simulink model "Sim_V1_scaling"  (R2018a)
settings: Solver=FixedStepAuto  StartTime=0.0  StopTime=tend  FixedStep=dt  MinStep=1e-3  RelTol=1e-3
values from neighbouring files (symbols this model uses):
  aref0 = a0+c*v0    [Init_Plots_Paper_V12.m]    (also in Init_Plots_Paper_V12_compare_high_low_fb.m; Init_Plots_Paper_V12_convergence_scaling.m; Sim_V1_MPC_step.mat = [0 0 0]; Sim_V1_MPC_step_base.mat = [0 0 0])
  dt = 1/1000    (= 0.001)    [Init_Plots_Paper_V12.m]    (also in Init_Plots_Paper_V12_compare_high_low_fb.m; Init_Plots_Paper_V12_convergence_scaling.m; Sim_V1_MPC_step.mat; Sim_V1_MPC_step_base.mat)
  dt_MPC = tau    (= 0.05)    [Init_Plots_Paper_V12.m]    (also in Init_Plots_Paper_V12_compare_high_low_fb.m; Init_Plots_Paper_V12_convergence_scaling.m; Sim_V1_MPC_step.mat; Sim_V1_MPC_step_base.mat)
  nconstr = 2*N+2    (= 102)    [Init_Plots_Paper_V12.m]    (also in Init_Plots_Paper_V12_compare_high_low_fb.m; Init_Plots_Paper_V12_convergence_scaling.m; Sim_V1_MPC_step.mat; Sim_V1_MPC_step_base.mat)
  p0 = [-10;5;3]    [Init_Plots_Paper_V12.m]    (also in Init_Plots_Paper_V12_compare_high_low_fb.m; Init_Plots_Paper_V12_convergence_scaling.m; Sim_V1_MPC_step.mat = [-10 5 3]; Sim_V1_MPC_step_base.mat = [-10 5 3])
  r30 = r30./norm(r30,2)    [Init_Plots_Paper_V12.m]    (also in Init_Plots_Paper_V12_compare_high_low_fb.m; Init_Plots_Paper_V12_convergence_scaling.m; Sim_V1_MPC_step.mat = [0 0 1]; Sim_V1_MPC_step_base.mat = [0 0 1])
  uMPC0 = [ux;uy;uz]    [Init_Plots_Paper_V12.m]    (also in Init_Plots_Paper_V12_compare_high_low_fb.m; Init_Plots_Paper_V12_convergence_scaling.m; Sim_V1_MPC_step.mat = [20 -60 -30]; Sim_V1_MPC_step_base.mat = [20 -60 -30])
  v0 = [-3;-1;2]    [Init_Plots_Paper_V12.m]    (also in Init_Plots_Paper_V12_compare_high_low_fb.m; Init_Plots_Paper_V12_convergence_scaling.m; Sim_V1_MPC_step.mat = [-3 -1 2]; Sim_V1_MPC_step_base.mat = [-3 -1 2])
libraries: dspmathops x2
settings Model: Creator=aandrien  LastModifiedBy=aandrien

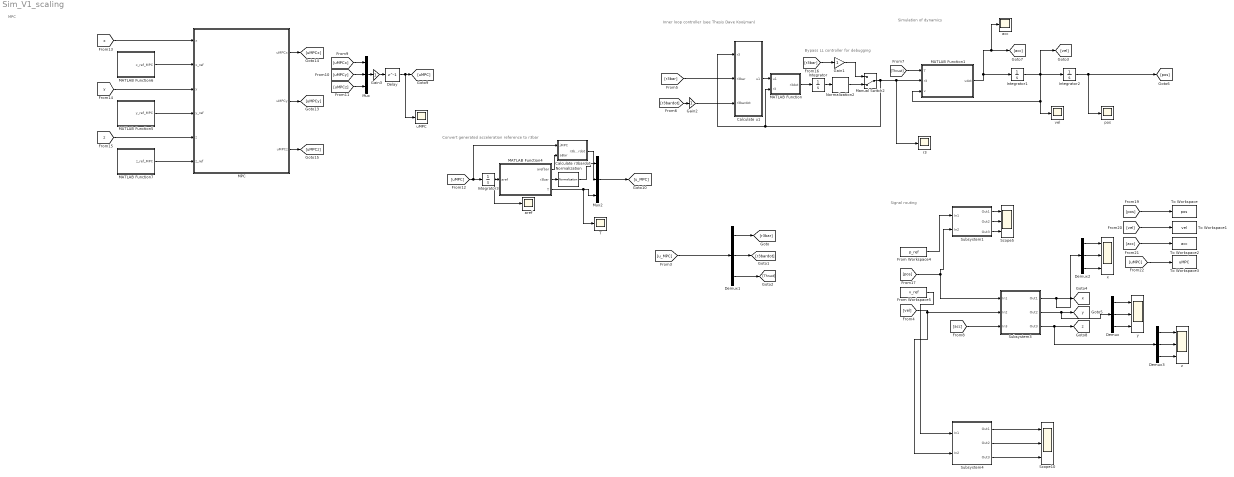
== system Sim_V1_scaling ==
  note: Inner loop controller (see Thesis Dave Kooijman)
  note: Bypass LL controller for debugging
  note: Simulation of dynamics
  note: MPC
  note: Signal routing
  note: Convert generated acceleration reference to r3bar
  Calculate r3bardot : MATLAB Function  TreatAsAtomicUnit=on
  Calculate u1 : MATLAB Function  TreatAsAtomicUnit=on
  Delay : Delay  DelayLength=1  InitialCondition=uMPC0  SampleTime=dt
  Demux : Demux  Outputs=3
  Demux1 : Demux  Outputs=[3,3,1]
  Demux2 : Demux  Outputs=3
  Demux3 : Demux  Outputs=3
  From Workspace4 : FromWorkspace  VariableName=p_ref  SampleTime=dt
  From Workspace5 : FromWorkspace  VariableName=v_ref  SampleTime=dt
  Gain1 : Gain
  Gain2 : Gain
  Gain3 : Gain
  Integrator : Integrator  InitialCondition=r30
  Integrator1 : Integrator  InitialCondition=v0
  Integrator2 : Integrator  InitialCondition=p0
  Integrator3 : Integrator  InitialCondition=aref0
  MATLAB Function : MATLAB Function  TreatAsAtomicUnit=on
  MATLAB Function1 : MATLAB Function  TreatAsAtomicUnit=on
  MATLAB Function4 : MATLAB Function  TreatAsAtomicUnit=on
  MATLAB Function5 : MATLAB Function  TreatAsAtomicUnit=on
      settings: MinAlgLoopOccurrences=on
  MATLAB Function6 : MATLAB Function  TreatAsAtomicUnit=on
      settings: MinAlgLoopOccurrences=on
  MATLAB Function7 : MATLAB Function  TreatAsAtomicUnit=on
  MPC : Subsystem
  Manual Switch2 : ManualSwitch  CurrentSetting=0
  Mux : Mux  Inputs=3
  Mux2 : Mux  Inputs=3
  Normalization : dspmathops/Normalization  NormType=2-norm  Bias=1e-10  NormOver=Each column  Dimension=1  roundingMode=Floor  overflowMode=off  accumDataTypeStr=Inherit: Same as product output  accumLastDataTypeStr=Inherit: Same as product output  outputDataTypeStr=Inherit: Same as product output  outputMin=[]  outputMax=[]  outputLastDataTypeStr=Inherit: Same as product output
      settings: SourceProductName=DSP System Toolbox
  Normalization2 : dspmathops/Normalization  NormType=2-norm  Bias=1e-10  NormOver=Each column  Dimension=1  roundingMode=Floor  overflowMode=off  accumDataTypeStr=Inherit: Same as product output  accumLastDataTypeStr=Inherit: Same as product output  outputDataTypeStr=Inherit: Same as product output  outputMin=[]  outputMax=[]  outputLastDataTypeStr=Inherit: Same as product output
      settings: SourceProductName=DSP System Toolbox
  Scope10 : Scope  NumInputPorts=3
  Scope5 : Scope  NumInputPorts=3
  Subsystem1 : Subsystem  mask{nInputs=2, nSize=3}
      mask prompts: nInputs "Number of Inputs"; nSize "Number of Outputs"
      mask init:
      | %% Input/output ports
      | inBlocks = find_system(gcb,...
      |     'LookUnderMasks','on',...
      |     'FollowLinks','on',...
      |     'BlockType','Inport');
      | 
      | outBlocks = find_system(gcb,...
      |     'LookUnderMasks','on',...
      |     'FollowLinks','on',...
      |     'BlockType','Outport');
      | 
      | demuxBlocks = find_system(gcb,...
      |     'LookUnderMasks','on',...
      |     'FollowLinks','on',...
      |     'BlockType','Demux');
      | 
      | muxBlocks = find_system(gcb,...
      |     'LookUnderMasks','on',...
      |     'FollowLinks','on',...
      |     'BlockType','Mux');
      | 
      | lines = find_system(gcb,...
      |     'LookUnderMasks','on',...
      |     'FollowLinks','on',...
      |     'FindAll','on',...
      |     'type','line');
      | 
      | if(size(inBlocks,1)~=nInputs || size(outBlocks,1)~=nSize) %check if number of input ports are as specfied
      |     delete_line(lines);
      |     delete_block(inBlocks); %delete all input ports
      |     delete_block(outBlocks); %delete all output ports
      |     delete_block(demuxBlocks);
      |     delete_block(muxBlocks);
      |     
      |     for k = 1:nInputs %add number of specified input ports
      |         add_block('built-in/Inport',[gcb,'/In',num2str(k)]); %add Input port
      |         set_param([gcb,'/In',num2str(k)],'position',[0,0+(k-1)*200,20,20+(k-1)*200]); %move input port for clarity
      |         %% Demux input ports
      |         add_block('simulink/Signal Routing/Demux',[gcb,'/Demux',num2str(k)]); %add demux
      |         set_param([gcb,'/Demux',num2str(k)],'position',[60,-60+(k-1)*200,65,80+(k-1)*200]); %move demux for clarity
      |         set_param([gcb,'/Demux',num2str(k)],'Outputs',num2str(nSize)) %set number of outputs from demux
      |         add_line(gcb,['In',num2str(k),'/1'],['Demux',num2str(k),'/1']) %connect input ports to demuxes
      |     end
      |     
      |     for k = 1:nSize %add number of specified output ports
      |         add_block('built-in/Outport',[gcb,'/Out',num2str(k)]);
      |         set_param([gcb,'/Out',num2str(k)],'position',[200,0+(k-1)*200,220,20+(k-1)*200]); %move output port for clarity
      |         %% Mux input ports
      |         add_block('simulink/Signal Routing/Mux',[gcb,'/Mux',num2str(k)]); %add demux
      |         set_param([gcb,'/Mux',num2str(k)],'position',[150,-60+(k-1)*200,155,80+(k-1)*200]); %move demux for clarity
      |         set_param([gcb,'/Mux',num2str(k)],'Inputs',num2str(nInputs)) %set number of inputs to mux
      |         add_line(gcb,['Mux',num2str(k),'/1'],['Out',num2str(k),'/1']) %connect muxes to output ports
      |     end
      |     
      |     %% Connect demuxes to muxes
      |     for ii = 1:nInputs
      |         for jj = 1:nSize
      |             add_line(gcb,['Demux',num2str(ii),'/',num2str(jj)],...
      |                 ['Mux',num2str(jj),'/',num2str(ii)],...
      |                 'autorouting','smart') %connect demuxes to muxes
      |         end
      |     end
      | end
  Subsystem3 : Subsystem  mask{nInputs=3, nSize=3}
      mask prompts: nInputs "Number of Inputs"; nSize "Number of Outputs"
      mask init: same as Sim_V1_scaling/Subsystem1
  Subsystem4 : Subsystem  mask{nInputs=2, nSize=3}
      mask prompts: nInputs "Number of Inputs"; nSize "Number of Outputs"
      mask init: same as Sim_V1_scaling/Subsystem1
  T : Scope
  To Workspace : ToWorkspace  VariableName=pos  SampleTime=-1
      settings: Save2DSignal=2-D array (concatenate along first dimension)
  To Workspace1 : ToWorkspace  VariableName=vel  SampleTime=-1
      settings: Save2DSignal=2-D array (concatenate along first dimension)
  To Workspace2 : ToWorkspace  VariableName=acc  SampleTime=-1
      settings: Save2DSignal=2-D array (concatenate along first dimension)
  To Workspace3 : ToWorkspace  VariableName=uMPC  SampleTime=-1
      settings: Save2DSignal=2-D array (concatenate along first dimension)
  acc : Scope
  aref : Scope
  pos : Scope
  r3 : Scope
  uMPC : Scope
  vel : Scope
  x : Scope  NumInputPorts=3
  y : Scope  NumInputPorts=3
  z : Scope  NumInputPorts=3
  tag scope: x=global, y=global, z=global
  wires:
  [Thrust] -> MATLAB Function1/1(T)
  [r3bardot] -> Gain2/1
  Calculate u1/1(u1) -> MATLAB Function/1(u1)
  MATLAB Function1/1(vdot) -> Integrator1/1, acc/1, [acc]
  Normalization2/1 -> Manual Switch2/2
  [r3bar] -> Gain1/1
  MATLAB Function/1(r3dot) -> Integrator/1
  [acc] -> Subsystem3/3(In3)
  Subsystem3/2(Out2) -> Demux/1, [y]
  [uMPCy] -> Mux/2
  Mux/1 -> Gain3/1
  [uMPC] -> Integrator3/1, Calculate r3bardot/1(jMPC)
  MATLAB Function4/1(arefbar) -> Calculate r3bardot/2(aBar)
  MATLAB Function4/3(T) -> T/1, Mux2/3
  Calculate r3bardot/1(r3bardot) -> Mux2/2
  MATLAB Function4/2(r3bar) -> Normalization/1
  Integrator3/1 -> aref/1, MATLAB Function4/1(aref)
  [uMPCx] -> Mux/1
  [uMPCz] -> Mux/3
  From Workspace4/1 -> Subsystem1/1(In1)
  [pos] -> Subsystem3/1(In1), Subsystem1/2(In2)
  Subsystem1/1(Out1) -> Scope5/1
  Subsystem1/2(Out2) -> Scope5/2
  Subsystem1/3(Out3) -> Scope5/3
  Gain1/1 -> Manual Switch2/1
  MPC/2(uMPCy) -> [uMPCy]
  Normalization/1 -> Mux2/1
  Integrator2/1 -> [pos], pos/1
  From Workspace5/1 -> Subsystem4/1(In1)
  [vel] -> Subsystem3/2(In2), Subsystem4/2(In2)
  Integrator/1 -> Normalization2/1
  MPC/1(uMPCx) -> [uMPCx]
  MPC/3(uMPCz) -> [uMPCz]
  Integrator1/1 -> vel/1, MATLAB Function1/3(v), [vel], Integrator2/1
  MATLAB Function5/1(y_ref_MPC) -> MPC/4(y_ref)
  MATLAB Function6/1(x_ref_MPC) -> MPC/2(x_ref)
  MATLAB Function7/1(z_ref_MPC) -> MPC/6(z_ref)
  Manual Switch2/1 -> MATLAB Function/2(r3), Calculate u1/1(r3), r3/1, MATLAB Function1/2(r3)
  [r3bar] -> Calculate u1/2(r3bar)
  Gain2/1 -> Calculate u1/3(r3bardot)
  Subsystem4/2(Out2) -> Scope10/2
  Subsystem4/1(Out1) -> Scope10/1
  Subsystem4/3(Out3) -> Scope10/3
  Demux/1 -> y/1
  Demux/2 -> y/2
  Demux/3 -> y/3
  [u_MPC] -> Demux1/1
  Demux1/3 -> [Thrust]
  Demux1/1 -> [r3bar]
  Demux1/2 -> [r3bardot]
  [pos] -> To Workspace/1
  [vel] -> To Workspace1/1
  [acc] -> To Workspace2/1
  [uMPC] -> To Workspace3/1
  Demux2/3 -> x/3
  Demux2/2 -> x/2
  Demux2/1 -> x/1
  Subsystem3/1(Out1) -> Demux2/1, [x]
  Demux3/3 -> z/3
  Demux3/1 -> z/1
  Subsystem3/3(Out3) -> Demux3/1, [z]
  Demux3/2 -> z/2
  [x] -> MPC/1(x)
  [y] -> MPC/3(y)
  [z] -> MPC/5(z)
  Mux2/1 -> [u_MPC]
  Gain3/1 -> Delay/1
  Delay/1 -> uMPC/1, [uMPC]

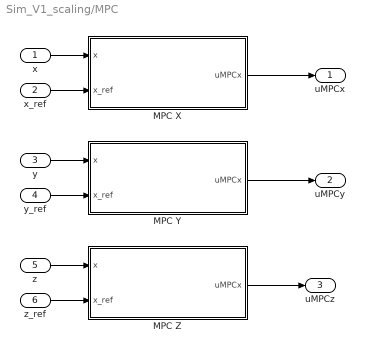
== system Sim_V1_scaling/MPC ==
  x : Inport
  x_ref : Inport  Port=2
  y : Inport  Port=3
  y_ref : Inport  Port=4
  z : Inport  Port=5
  z_ref : Inport  Port=6
  MPC X : Subsystem
  MPC Y : Subsystem
  MPC Z : Subsystem
  uMPCx : Outport
  uMPCy : Outport  Port=2
  uMPCz : Outport  Port=3
  wires:
  MPC X/1(uMPCx) -> uMPCx/1
  x/1 -> MPC X/1(x)
  y/1 -> MPC Y/1(x)
  z/1 -> MPC Z/1(x)
  y_ref/1 -> MPC Y/2(x_ref)
  x_ref/1 -> MPC X/2(x_ref)
  z_ref/1 -> MPC Z/2(x_ref)
  MPC Z/1(uMPCx) -> uMPCz/1
  MPC Y/1(uMPCx) -> uMPCy/1

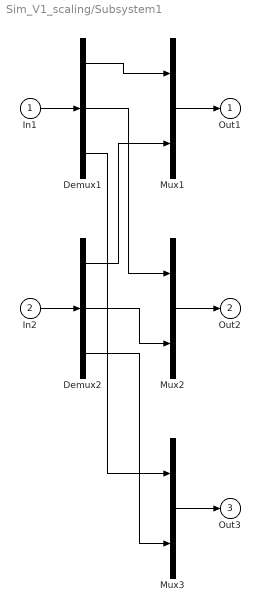
== system Sim_V1_scaling/Subsystem1 ==
  In1 : Inport
  In2 : Inport  Port=2
  Demux1 : Demux  Outputs=3
  Demux2 : Demux  Outputs=3
  Mux1 : Mux  Inputs=2
  Mux2 : Mux  Inputs=2
  Mux3 : Mux  Inputs=2
  Out1 : Outport
  Out2 : Outport  Port=2
  Out3 : Outport  Port=3
  wires:
  In1/1 -> Demux1/1
  In2/1 -> Demux2/1
  Mux1/1 -> Out1/1
  Mux2/1 -> Out2/1
  Mux3/1 -> Out3/1
  Demux1/1 -> Mux1/1
  Demux1/2 -> Mux2/1
  Demux1/3 -> Mux3/1
  Demux2/1 -> Mux1/2
  Demux2/2 -> Mux2/2
  Demux2/3 -> Mux3/2

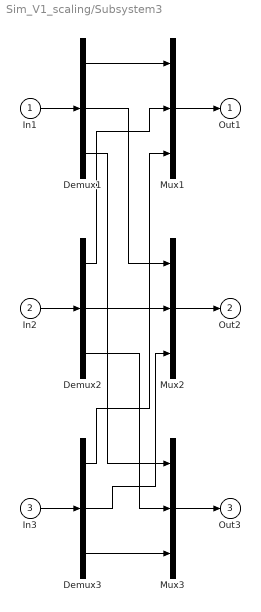
== system Sim_V1_scaling/Subsystem3 ==
  In1 : Inport
  In2 : Inport  Port=2
  In3 : Inport  Port=3
  Demux1 : Demux  Outputs=3
  Demux2 : Demux  Outputs=3
  Demux3 : Demux  Outputs=3
  Mux1 : Mux  Inputs=3
  Mux2 : Mux  Inputs=3
  Mux3 : Mux  Inputs=3
  Out1 : Outport
  Out2 : Outport  Port=2
  Out3 : Outport  Port=3
  wires:
  In1/1 -> Demux1/1
  In2/1 -> Demux2/1
  In3/1 -> Demux3/1
  Mux1/1 -> Out1/1
  Mux2/1 -> Out2/1
  Mux3/1 -> Out3/1
  Demux1/1 -> Mux1/1
  Demux1/2 -> Mux2/1
  Demux1/3 -> Mux3/1
  Demux2/1 -> Mux1/2
  Demux2/2 -> Mux2/2
  Demux2/3 -> Mux3/2
  Demux3/1 -> Mux1/3
  Demux3/2 -> Mux2/3
  Demux3/3 -> Mux3/3

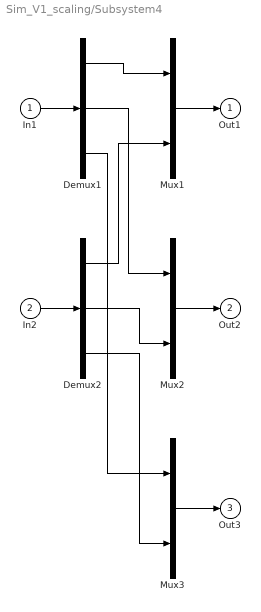
== system Sim_V1_scaling/Subsystem4 ==
  In1 : Inport
  In2 : Inport  Port=2
  Demux1 : Demux  Outputs=3
  Demux2 : Demux  Outputs=3
  Mux1 : Mux  Inputs=2
  Mux2 : Mux  Inputs=2
  Mux3 : Mux  Inputs=2
  Out1 : Outport
  Out2 : Outport  Port=2
  Out3 : Outport  Port=3
  wires:
  In1/1 -> Demux1/1
  In2/1 -> Demux2/1
  Mux1/1 -> Out1/1
  Mux2/1 -> Out2/1
  Mux3/1 -> Out3/1
  Demux1/1 -> Mux1/1
  Demux1/2 -> Mux2/1
  Demux1/3 -> Mux3/1
  Demux2/1 -> Mux1/2
  Demux2/2 -> Mux2/2
  Demux2/3 -> Mux3/2

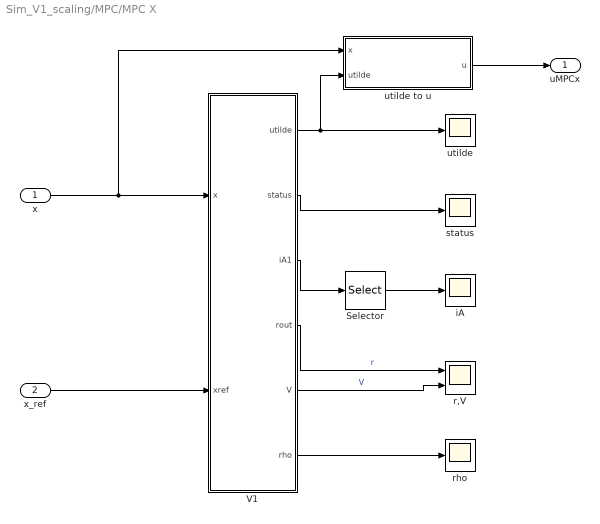
== system Sim_V1_scaling/MPC/MPC X ==
  x : Inport
  x_ref : Inport  Port=2
  Selector : Selector  InputPortWidth=nconstr  IndexOptions=Index vector (dialog)  Indices=nconstr-1:nconstr  OutputSizes=1
  V1 : MATLAB Function  TreatAsAtomicUnit=on  SystemSampleTime=dt_MPC
  iA : Scope
  r,V : Scope  NumInputPorts=2
  rho : Scope
  status : Scope
  utilde : Scope
  utilde to u : MATLAB Function  TreatAsAtomicUnit=on
  uMPCx : Outport
  wires:
  V1/4(rout) -> r,V/1  "r"
  V1/5(V) -> r,V/2  "V"
  x/1 -> V1/1(x), utilde to u/1(x)
  x_ref/1 -> V1/2(xref)
  V1/1(utilde) -> utilde/1, utilde to u/2(utilde)
  V1/2(status) -> status/1
  utilde to u/1(u) -> uMPCx/1
  V1/3(iA1) -> Selector/1
  Selector/1 -> iA/1
  V1/6(rho) -> rho/1

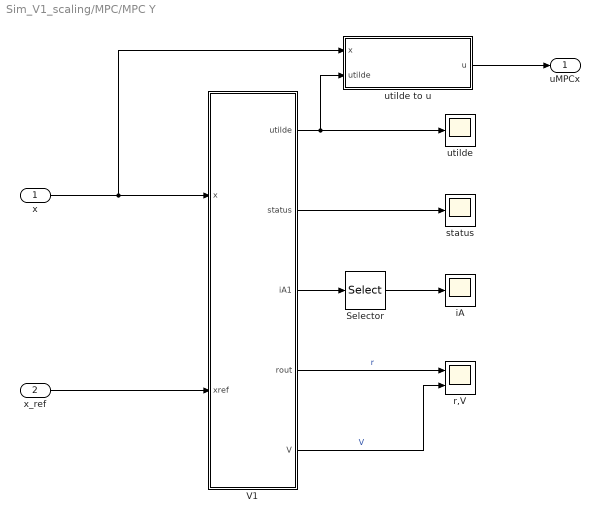
== system Sim_V1_scaling/MPC/MPC Y ==
  x : Inport
  x_ref : Inport  Port=2
  Selector : Selector  InputPortWidth=nconstr  IndexOptions=Index vector (dialog)  Indices=nconstr-1:nconstr  OutputSizes=1
  V1 : MATLAB Function  TreatAsAtomicUnit=on  SystemSampleTime=dt_MPC
  iA : Scope
  r,V : Scope  NumInputPorts=2
  status : Scope
  utilde : Scope
  utilde to u : MATLAB Function  TreatAsAtomicUnit=on
  uMPCx : Outport
  wires:
  Selector/1 -> iA/1
  V1/3(iA1) -> Selector/1
  utilde to u/1(u) -> uMPCx/1
  V1/2(status) -> status/1
  V1/1(utilde) -> utilde to u/2(utilde), utilde/1
  x_ref/1 -> V1/2(xref)
  x/1 -> utilde to u/1(x), V1/1(x)
  V1/5(V) -> r,V/2  "V"
  V1/4(rout) -> r,V/1  "r"

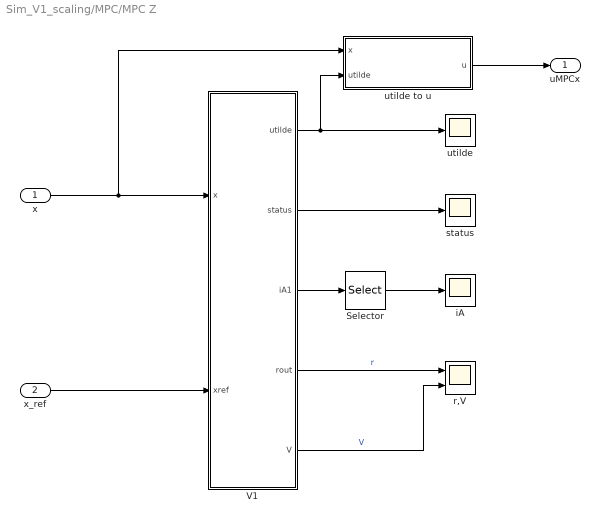
== system Sim_V1_scaling/MPC/MPC Z ==
  x : Inport
  x_ref : Inport  Port=2
  Selector : Selector  InputPortWidth=nconstr  IndexOptions=Index vector (dialog)  Indices=nconstr-1:nconstr  OutputSizes=1
  V1 : MATLAB Function  TreatAsAtomicUnit=on  SystemSampleTime=dt_MPC
  iA : Scope
  r,V : Scope  NumInputPorts=2
  status : Scope
  utilde : Scope
  utilde to u : MATLAB Function  TreatAsAtomicUnit=on
  uMPCx : Outport
  wires:
  V1/4(rout) -> r,V/1  "r"
  V1/5(V) -> r,V/2  "V"
  x/1 -> V1/1(x), utilde to u/1(x)
  x_ref/1 -> V1/2(xref)
  V1/1(utilde) -> utilde/1, utilde to u/2(utilde)
  V1/2(status) -> status/1
  utilde to u/1(u) -> uMPCx/1
  V1/3(iA1) -> Selector/1
  Selector/1 -> iA/1

== matlab function Sim_V1_scaling/MPC/MPC Y/V1 ==
  settings: updateMethod=DISCRETE  sampleTime=dt_MPC
  data: utilde output; status output; iA1 output; x input size=[3 1]; xref input; mpc_params parameter; rout output; V output
function [utilde, status, iA1, rout, V] = MPC(x, xref, mpc_params)
%#codegen
%% Retrieve parameters
Atil = mpc_params.Atil;
B = mpc_params.B;
Q = mpc_params.Q;
R = mpc_params.R;
N = mpc_params.N;
Deltatil = mpc_params.Deltatil;
Delta = mpc_params.Delta;
base = mpc_params.base;

%% Calculate P_epsilon (solution to DARE with scheduling epsilon)
r = 0.99;
% P = dare(Atil,B,r*Q,R);
P = 1000*eye(3);
for k = 1:500
    P = Atil'*P*Atil+r*Q-Atil'*P*B*inv(R+B'*P*B)*B'*P*Atil;
end
while(x'*P*x*trace(P)>R*Delta^2/(2*trace(B*B')))
    r = 0.99*r;
    for k = 1:100
        P = Atil'*P*Atil+r*Q-Atil'*P*B*inv(R+B'*P*B)*B'*P*Atil;
    end
end
Pout = P;
rout = r;

F = -inv(B'*P*B+R)*B'*P*Atil;
S = sign(R*F*x);

%% Inequality constraints
Aineq = [-eye(N); % U_{l|k} <= Delta
    eye(N); % -Delta <= U_{l|k}
    S*[1,zeros(1,N-1)]; % 0<= sign(R*F*x)[u_{0|k}-F*x]
    -S*B'*P*B*[1,zeros(1,N-1)]]; % 0<= sign(R*F*x)(2*R*F-B'*P*B*[u_{0|k}-F*x])

bineq = [-Deltatil; % U_{l|k} <= Delta
    -Deltatil; % -Delta <= U_{l|k}
    S*F*x; % 0<= sign(RFx)[u_{0|k}-Fx]
    -2*S*R*F*x-S*B'*P*B*F*x]; % 0<= sign(R*F*x)(2*R*F-B'*P*B*[u_{0|k}-F*x])

%% Equality constraints
Aeq = []; % no equality constraints
beq = zeros(0,1); % no equality constraints

[uMPC, status, iA1] = mpcqpsolver(mpc_params.Linv, mpc_params.f*(mpc_params.Ftil*x-xref), Aineq, bineq, Aeq, beq, false(size(bineq,1),1), mpc_params.opt);

if(status<= 0)
    utilde = F*x;
else
    utilde = uMPC(1);
end
if(base)
    utilde = F*x;
end
V = x'*Pout*x;

== matlab function Sim_V1_scaling/MATLAB Function1 ==
  data: T input; vdot output; r3 input; v input; quad_params parameter
function vdot = velocity_dynamics(T,r3,v,quad_params)

fd = -quad_params.c*v;
vdot = [0;0;quad_params.g]+(fd-T*r3)/quad_params.m;

== matlab function Sim_V1_scaling/Calculate u1 ==
  data: r3 input; r3bar input; u1 output; r3bardot input
function u1 = fcn(r3,r3bar,r3bardot)
k1 = 500;

s = sqrt(1-(r3'*r3bar)^2);
% theta = (cross(r3,r3bar)*transpose(cross(r3,r3bar))-...
%         (eye(3)-r3*transpose(r3))*r3bar*transpose(r3))/s^2;

theta = (cross(r3,r3bar)*transpose(cross(r3,r3bar))-...
        (eye(3)-r3*transpose(r3))*r3bar*transpose(r3));

% if r3 == r3bar
%     uff = r3bardot;
% elseif r3 == -r3bar
%     uff = -r3bardot;
% else
%     uff = -k1*(r3bar-r3);
% end
% % theta*r3bardot
% if r3'*r3bar >= 0
%     ufb = k1*r3bar;
% else
%     ufb = k1*r3bar/s;
% end
% 
% u1 = uff;

if r3 == r3bar
    u1 = r3bardot;
else
    u1 = theta*r3bardot-k1*(r3bar-r3);
end
u1 = -u1;

== matlab function Sim_V1_scaling/MATLAB Function ==
  data: u1 input; r3dot output; r3 input
function r3dot = fcn(u1,r3)

r3dot = (eye(3)-r3*transpose(r3))*u1;

== matlab function Sim_V1_scaling/MPC/MPC Y/utilde to u ==
  data: x input; utilde input; u output; mpc_params parameter
function u = input_transf(x, utilde,  mpc_params)
c7 = mpc_params.c7;

u = utilde-x(3)/c7;

== matlab function Sim_V1_scaling/MPC/MPC X/V1 ==
  settings: updateMethod=DISCRETE  sampleTime=dt_MPC
  data: utilde output; status output; iA1 output; x input size=[3 1]; xref input; mpc_params parameter; rout output; V output; rho output
function [utilde, status, iA1, rout, V, rho] = MPC(x, xref, mpc_params)
%#codegen
%% Retrieve parameters
Atil = mpc_params.Atil;
B = mpc_params.Btil;
Q = mpc_params.Q;
R = mpc_params.R;
N = mpc_params.N;
Deltatil = mpc_params.Deltatil;
Delta = mpc_params.Delta;
alf = mpc_params.alf;
scale = mpc_params.scale;
base = mpc_params.base;
high = mpc_params.high;

%% Calculate P_epsilon (solution to DARE with scheduling epsilon)
r = 0.99;
% P = dare(Atil,B,r*Q,R);
P = 1000*eye(3);
for k = 1:500
    P = Atil'*P*Atil+r*Q-Atil'*P*B*inv(R+B'*P*B)*B'*P*Atil;
end
while(x'*P*x*trace(P)>R*Delta^2/(2*trace(B*B')))
    r = 0.99*r;
    for k = 1:100
        P = Atil'*P*Atil+r*Q-Atil'*P*B*inv(R+B'*P*B)*B'*P*Atil;
    end
end
Pout = P;
rout = r;

F = -inv(B'*P*B+R)*B'*P*Atil;
S = sign(R*F*x);

%% Inequality constraints
Aineq = [-eye(N); % U_{l|k} <= Delta
    eye(N); % -Delta <= U_{l|k}
    S*[1,zeros(1,N-1)]; % 0<= sign(R*F*x)[u_{0|k}-F*x]
    -S*B'*P*B*[1,zeros(1,N-1)]]; % 0<= sign(R*F*x)(2*R*F-B'*P*B*[u_{0|k}-F*x])

bineq = [-Deltatil.*alf; % U_{l|k} <= Delta
    -Deltatil.*alf; % -Delta <= U_{l|k}
    S*F*x; % 0<= sign(RFx)[u_{0|k}-Fx]
    -2*S*R*F*x-S*B'*P*B*F*x]; % 0<= sign(R*F*x)(2*R*F-B'*P*B*[u_{0|k}-F*x])

%% Equality constraints
Aeq = []; % no equality constraints
beq = zeros(0,1); % no equality constraints

[uMPC, status, iA1] = mpcqpsolver(mpc_params.Linv, mpc_params.f*(mpc_params.Ftil*x-xref), Aineq, bineq, Aeq, beq, false(size(bineq,1),1), mpc_params.opt);
rho = 0;
if(status<= 0)
    utilde = F*x;
else
    utilde = uMPC(1);
end
if(base)
    if(high)
        rho = 0.9*R^2*2/norm(B'*P*B);
        utilde = F*x+rho*F*x;
    else
        utilde = F*x;
    end
end
if(scale)
    utilde = utilde/alf;
end
V = x'*Pout*x;

== matlab function Sim_V1_scaling/MPC/MPC X/utilde to u ==
  data: x input; utilde input; u output; mpc_params parameter
function u = input_transf(x, utilde,  mpc_params)
c7 = mpc_params.c7;

u = utilde-x(3)/c7;

== matlab function Sim_V1_scaling/MPC/MPC Z/V1 ==
  settings: updateMethod=DISCRETE  sampleTime=dt_MPC
  data: utilde output; status output; iA1 output; x input size=[3 1]; xref input; mpc_params parameter; rout output; V output
function [utilde, status, iA1, rout, V] = MPC(x, xref, mpc_params)
%#codegen
%% Retrieve parameters
Atil = mpc_params.Atil;
B = mpc_params.B;
Q = mpc_params.Q;
R = mpc_params.R;
N = mpc_params.N;
Deltatil = mpc_params.Deltatil;
Delta = mpc_params.Delta;
base = mpc_params.base;

%% Calculate P_epsilon (solution to DARE with scheduling epsilon)
r = 0.99;
% P = dare(Atil,B,r*Q,R);
P = 1000*eye(3);
for k = 1:500
    P = Atil'*P*Atil+r*Q-Atil'*P*B*inv(R+B'*P*B)*B'*P*Atil;
end
while(x'*P*x*trace(P)>R*Delta^2/(2*trace(B*B')))
    r = 0.99*r;
    for k = 1:100
        P = Atil'*P*Atil+r*Q-Atil'*P*B*inv(R+B'*P*B)*B'*P*Atil;
    end
end
Pout = P;
rout = r;

F = -inv(B'*P*B+R)*B'*P*Atil;
S = sign(R*F*x);

%% Inequality constraints
Aineq = [-eye(N); % U_{l|k} <= Delta
    eye(N); % -Delta <= U_{l|k}
    S*[1,zeros(1,N-1)]; % 0<= sign(R*F*x)[u_{0|k}-F*x]
    -S*B'*P*B*[1,zeros(1,N-1)]]; % 0<= sign(R*F*x)(2*R*F-B'*P*B*[u_{0|k}-F*x])

bineq = [-Deltatil; % U_{l|k} <= Delta
    -Deltatil; % -Delta <= U_{l|k}
    S*F*x; % 0<= sign(RFx)[u_{0|k}-Fx]
    -2*S*R*F*x-S*B'*P*B*F*x]; % 0<= sign(R*F*x)(2*R*F-B'*P*B*[u_{0|k}-F*x])

%% Equality constraints
Aeq = []; % no equality constraints
beq = zeros(0,1); % no equality constraints

[uMPC, status, iA1] = mpcqpsolver(mpc_params.Linv, mpc_params.f*(mpc_params.Ftil*x-xref), Aineq, bineq, Aeq, beq, false(size(bineq,1),1), mpc_params.opt);

if(status<= 0)
    utilde = F*x;
else
    utilde = uMPC(1);
end
if(base)
    utilde = F*x;
end
V = x'*Pout*x;

== matlab function Sim_V1_scaling/MPC/MPC Z/utilde to u ==
  data: x input; utilde input; u output; mpc_params parameter
function u = input_transf(x, utilde,  mpc_params)
c7 = mpc_params.c7;

u = utilde-x(3)/c7;

== matlab function Sim_V1_scaling/MATLAB Function5 ==
  settings: updateMethod=DISCRETE  sampleTime=dt
  data: y_ref_MPC output; mpc_params parameter
function y_ref_MPC = MPC_ref_gen(mpc_params)
persistent cnt

if(isempty(cnt))
    cnt = 1;
end

% y_ref_MPC = mpc_params.y_ref(1+(cnt-1)*3:(cnt-1)*3+(mpc_params.N+1)*3,1);
if((cnt-1)*3+(mpc_params.N+1)*3>=size(mpc_params.y_ref,1))
    y_ref_MPC = zeros((mpc_params.N+1)*3,1);
else
    y_ref_MPC = mpc_params.y_ref(1+(cnt-1)*3:(cnt-1)*3+(mpc_params.N+1)*3,1);
end
cnt = cnt+1;

== matlab function Sim_V1_scaling/MATLAB Function6 ==
  settings: updateMethod=DISCRETE  sampleTime=dt_MPC
  data: x_ref_MPC output; mpc_params parameter
function x_ref_MPC = MPC_ref_gen(mpc_params)
persistent cnt

if(isempty(cnt))
    cnt = 1;
end


if((cnt-1)*3+(mpc_params.N+1)*3>=size(mpc_params.x_ref,1))
    x_ref_MPC = zeros((mpc_params.N+1)*3,1);
else
    x_ref_MPC = mpc_params.x_ref(1+(cnt-1)*3:(cnt-1)*3+(mpc_params.N+1)*3,1);
end
cnt = cnt+1;

== matlab function Sim_V1_scaling/MATLAB Function4 ==
  data: arefbar output; aref input; r3bar output; quad_params parameter; T output
function [arefbar,r3bar,T] = calc_ref_low_level(aref,quad_params)

% arefbar = -[0;0;quad_params.g]+aref;
arefbar = [0;0;quad_params.g]-aref;
r3bar = arefbar;

T = quad_params.m*norm(arefbar,2);

== matlab function Sim_V1_scaling/Calculate r3bardot ==
  data: jMPC input; r3bardot output; aBar input
function r3bardot = fcn(jMPC,aBar)

r3bar = aBar./norm(aBar,2);

num = jMPC.*norm(aBar,2)-r3bar.*(cross(aBar,jMPC)); 
den = norm(aBar,2)^2;




r3bardot = num./den;

== matlab function Sim_V1_scaling/MATLAB Function7 ==
  settings: updateMethod=DISCRETE  sampleTime=dt
  data: z_ref_MPC output; mpc_params parameter
function z_ref_MPC = MPC_ref_gen(mpc_params)
persistent cnt

if(isempty(cnt))
    cnt = 1;
end

if((cnt-1)*3+(mpc_params.N+1)*3>=size(mpc_params.z_ref,1))
    z_ref_MPC = zeros((mpc_params.N+1)*3,1);
else
    z_ref_MPC = mpc_params.z_ref(1+(cnt-1)*3:(cnt-1)*3+(mpc_params.N+1)*3,1);
end
cnt = cnt+1;
